simulink model "ObserverSimulation"  (R2025b)
settings: Solver=VariableStepAuto  StartTime=0.0  StopTime=10.0  RelTol=1e-3
values from neighbouring files (symbols this model uses):
  A_plant = [ ... (first row only)    [params.m]
  Aobs = Ad - L*Cd    [params.m]
  B_plant = [ ... (first row only)    [params.m]
  Bobs = [Bd, L]    [params.m]
  C_plant = [1 0 0; 0 1 0]    [params.m]
  Cobs = eye(4)    [params.m]
  D_plant = zeros(2,2)    [params.m]
  Dobs = zeros(4,3)    [params.m]
  Ki_current = Ra * 500    (= 516.05)    [params.m]
  Kp_current = La * 500    (= 0.25275)    [params.m]
  Kt_nominal = 0.754    [params.m]
  Ts = 200e-6    (= 0.0002)    [params.m]
undefined symbols (not defined in the file or in its folder): lpf_den, lpf_num
libraries: slpidlib x1
settings Model: Creator=atuly  LastModifiedBy=atuly

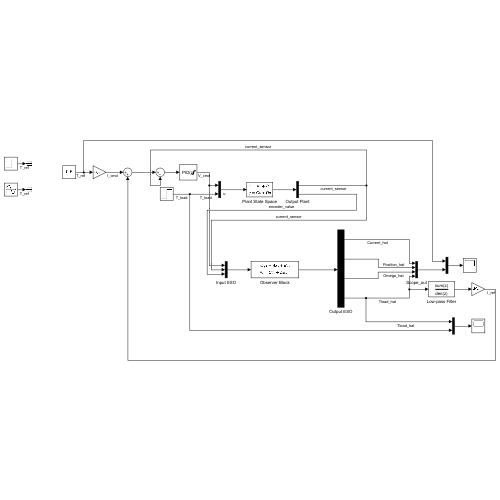
[thumbnail: Simulink's stored preview of the top-level diagram]
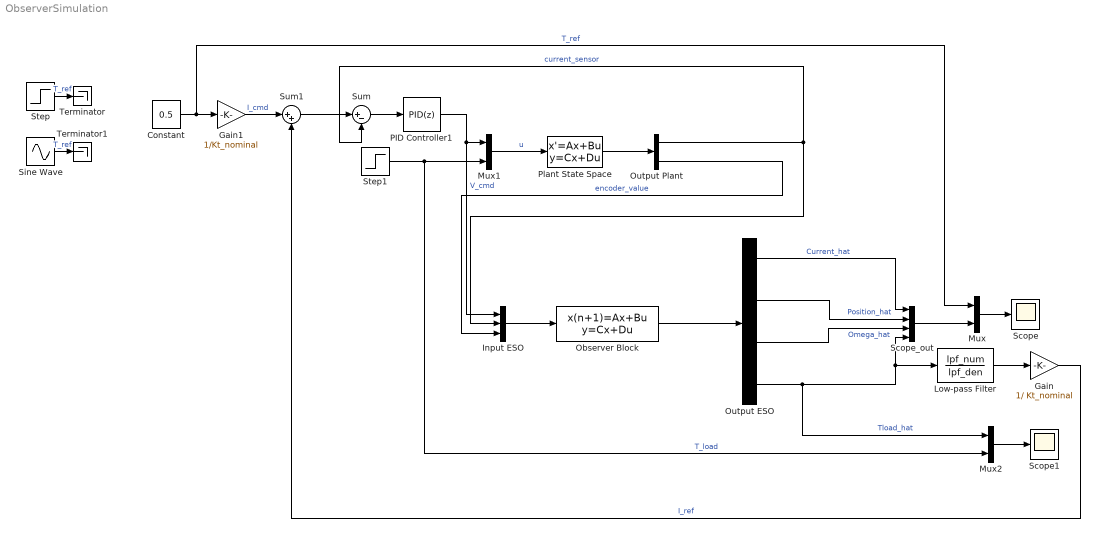
== system ObserverSimulation ==
  Constant : Constant  Value=0.5
  Gain : Gain  Gain=1/ Kt_nominal
  Gain1 : Gain  Gain=1/Kt_nominal
  Input ESO : Mux  Inputs=3
  Low-pass Filter : DiscreteFilter  Numerator=lpf_num  Denominator=lpf_den  FilterStructure=Direct form I
  Mux : Mux  Inputs=2
  Mux1 : Mux  Inputs=2
  Mux2 : Mux  Inputs=2
  Observer Block : DiscreteStateSpace  A=Aobs  B=Bobs  C=Cobs  D=Dobs  SampleTime=Ts
  Output ESO : Demux
  Output Plant : Demux  Outputs=2
  PID Controller1 : slpidlib/PID Controller  Controller=PID  Form=Parallel  TimeDomain=Discrete-time  UseExternalTs=off  SampleTime=Ts  IntegratorMethod=Forward Euler  FilterMethod=Forward Euler  ControllerParametersSource=internal  P=Kp_current  I=Ki_current  UseKiTs=off  D=0  UseExternalDerivativeSource=off  N=100  UseFilter=on  TunerSelectOption=Transfer Function Based (PID Tuner App)  InitialConditionSource=internal  InitialConditionForIntegrator=0  InitialConditionForFilter=0  DifferentiatorICPrevScaledInput=0  ExternalReset=none  TrackingMode=off  Kt=1  LimitOutput=on  SatLimitsSource=internal  UpperSaturationLimit=12.6  LowerSaturationLimit=-12.6  LinearizeAsGain=on  AntiWindupMode=none  Kb=1  LimitIntegrator=off  UpperIntegratorSaturationLimit=inf  LowerIntegratorSaturationLimit=-inf  POutMin=[]  POutMax=[]  IOutMin=[]  IOutMax=[]  DOutMin=[]  DOutMax=[]  NOutMin=[]  NOutMax=[]  SumOutMin=[]  SumOutMax=[]  SaturationOutMin=[]  SaturationOutMax=[]  PParamMin=[]  PParamMax=[]  IParamMin=[]  IParamMax=[]  DParamMin=[]  DParamMax=[]  NParamMin=[]  NParamMax=[]  KbParamMin=[]  KbParamMax=[]  KtParamMin=[]  KtParamMax=[]  KbOutMin=[]  KbOutMax=[]  KtOutMin=[]  KtOutMax=[]  IntegratorOutMin=[]  IntegratorOutMax=[]  FilterOutMin=[]  FilterOutMax=[]  SumI1OutMin=[]  SumI1OutMax=[]  SumI2OutMin=[]  SumI2OutMax=[]  SumI3OutMin=[]  SumI3OutMax=[]  SumI4OutMin=[]  SumI4OutMax=[]  SumDOutMin=[]  SumDOutMax=[]  DifferentiatorOutMin=[]  DifferentiatorOutMax=[]  FilterDiffOutCoefMin=[]  FilterDiffOutCoefMax=[]  ReciprocalOutMin=[]  ReciprocalOutMax=[]  SumDenOutMin=[]  SumDenOutMax=[]  SumNumOutMin=[]  SumNumOutMax=[]  DivideOutMin=[]  DivideOutMax=[]  UdiffTsProdOutMin=[]  UdiffTsProdOutMax=[]  NTsProdOutMin=[]  NTsProdOutMax=[]  UintegralTsProdOutMin=[]  UintegralTsProdOutMax=[]  UngainTsProdOutMin=[]  UngainTsProdOutMax=[]  ClampingZeroOutDataTypeStr=Inherit: Inherit via back propagation  ClampingZeroOutMin=[]  ClampingZeroOutMax=[]  FilterDenConstantOutDataTypeStr=Inherit: Inherit via back propagation  FilterDenConstantOutMin=[]  FilterDenConstantOutMax=[]  PCopyOutDataTypeStr=Inherit: Inherit via back propagation  PCopyOutMin=[]  PCopyOutMax=[]  NCopyOutDataTypeStr=Inherit: Inherit via back propagation  NCopyOutMin=[]  NCopyOutMax=[]  IntegratorContinuousStateAttributes=''  IntegratorStateMustResolveToSignalObject=off  IntegratorRTWStateStorageClass=Auto  FilterContinuousStateAttributes=''  FilterStateMustResolveToSignalObject=off  FilterRTWStateStorageClass=Auto  ParallelPVariant=InternalParameters  IdealPVariant=Disabled  IVariant=InternalParameters  DVariant=InternalParameters  IntegratorVariant=Discrete  SatVariant=Enabled  AWVariant=Passthrough  PCopyVariant=Disabled  TRVariant=Disabled  FdbkBlocksVariant=Forward  IdealPFdbkVariant=Disabled  SatFdbkVariant=Disabled  DerivativeFilterVariant=ForwardEulerFilter  NVariant=InternalParameters  NCopyVariant=Disabled  FilterICVariant=InternalICsFilter  IntegratorICVariant=InternalICs  ExternalResetVariant=Disabled  TRSumVariant=Passthrough  SumFdbkVariant=Disabled  SumVariant=Sum_PID  TsampFilterVariant=InternalTs  TsampNgainVariant=Passthrough  TsampIntegralVariant=Disabled_SignalSpec  ExternalSaturationOutDataTypeStr=Inherit: Same as second input  DerivativeSourceVariant=ErrorSignal  PreIntVariant=InternalPreInt
  Plant State Space : StateSpace  A=A_plant  B=B_plant  C=C_plant  D=D_plant  InitialCondition=[0,0,0]  ParameterTunability=Unconstrained
  Scope : Scope
      settings: ActiveDisplayYMinimum=-60.866535363223761  ActiveDisplayYMaximum=109.0682659415113
  Scope1 : Scope
      settings: ActiveDisplayYMinimum=-1.8599471641906211  ActiveDisplayYMaximum=4.1327435809656645
  Scope_out : Mux
  Sine Wave : Sin  Frequency=62  SampleTime=0
  Step : Step  SampleTime=Ts
  Step1 : Step  Time=3  After=1.3  SampleTime=Ts
  Sum : Sum  Inputs=|+-
  Sum1 : Sum  Inputs=|++
  Terminator : Terminator
  Terminator1 : Terminator
  wires:
  Output Plant/2 -> Input ESO/3  "encoder_value"
  Plant State Space/1 -> Output Plant/1
  Output Plant/1 -> Input ESO/2, Sum/2  "current_sensor"
  Mux1/1 -> Plant State Space/1  "u"
  Input ESO/1 -> Observer Block/1
  Observer Block/1 -> Output ESO/1
  Output ESO/1 -> Scope_out/1  "Current_hat"
  Output ESO/2 -> Scope_out/2  "Position_hat"
  Output ESO/3 -> Scope_out/3  "Omega_hat"
  Scope_out/1 -> Mux/2
  Output ESO/4 -> Mux2/1, Low-pass Filter/1, Scope_out/4  "Tload_hat"
  Mux2/1 -> Scope1/1
  Step1/1 -> Mux2/2, Mux1/2  "T_load"
  Low-pass Filter/1 -> Gain/1
  PID Controller1/1 -> Input ESO/1, Mux1/1  "V_cmd"
  Gain1/1 -> Sum1/1  "I_cmd"
  Constant/1 -> Mux/1, Gain1/1  "T_ref"
  Gain/1 -> Sum1/2  "I_ref"
  Sum1/1 -> Sum/1
  Sum/1 -> PID Controller1/1
  Step/1 -> Terminator/1  "T_ref"
  Sine Wave/1 -> Terminator1/1  "T_ref"
  Mux/1 -> Scope/1
